simulink model "project_2023_12_11_P46"  (R2021b)
settings: Solver=ode5  StartTime=0.0  StopTime=500  FixedStep=0.01  RelTol=1e-3
values from neighbouring files (symbols this model uses):
  c1 = 1    [project_2023_12_11_P46_1.m]
  c2 = 1    [project_2023_12_11_P46_1.m]
  g = 9.8    [project_2023_12_11_P46_1.m]
  m = 70    [project_2023_12_11_P46_1.m]
undefined symbols (not defined in the file or in its folder): k
settings Model: Creator=Administrator  LastModifiedBy=yingguang wang
settings SolverCC: AlgebraicLoopSolver=TrustRegion
settings DataIOCC: SaveFormat=Array  ReturnWorkspaceOutputs=off  TimeSaveName=t  OutputSaveName=y
settings DebuggingCC: SFMachineParentedDataDiag=warning  ArithmeticOperatorsInVariantConditions=warning
settings SFSimCC: SimUseLocalCustomCode=off  CustomCodeUndefinedFunction=UseInterfaceOnly
settings RTWCC: RTWUseLocalCustomCode=off

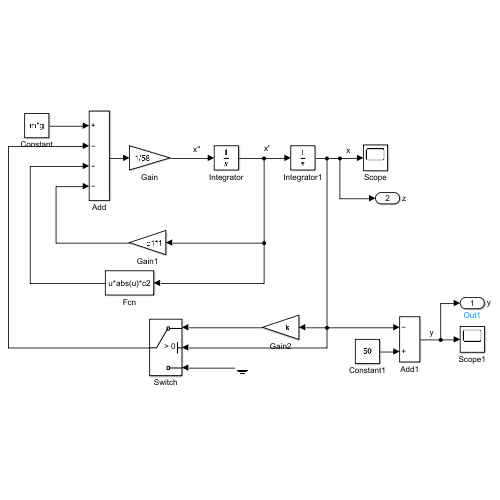
[thumbnail: Simulink's stored preview of the top-level diagram]
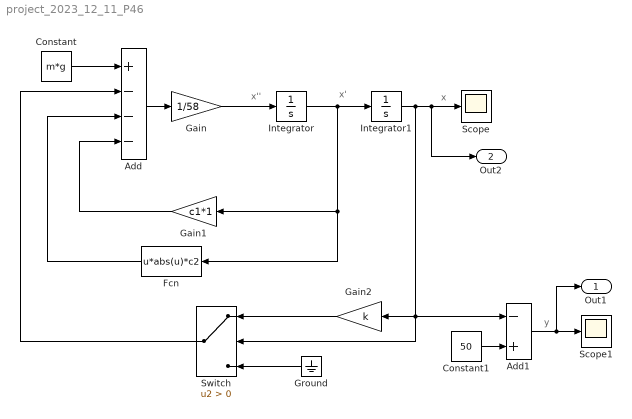
== system project_2023_12_11_P46 ==
  note: x'
  note: x''
  note: x
  note: y
  Add : Sum  Inputs=+---
  Add1 : Sum  Inputs=-+
  Constant : Constant  Value=m*g
  Constant1 : Constant  Value=50
  Fcn : Fcn  Expr=u*abs(u)*c2
  Gain : Gain  Gain=1/58
  Gain1 : Gain  Gain=c1*1
  Gain2 : Gain  Gain=k
  Ground : Ground
  Integrator : Integrator
  Integrator1 : Integrator  InitialCondition=-30
  Scope : Scope
  Scope1 : Scope
  Switch : Switch  Criteria=u2 > Threshold
  Out1 : Outport  SignalName=y  VectorParamsAs1DForOutWhenUnconnected=off
  Out2 : Outport  Port=2  SignalName=z  VectorParamsAs1DForOutWhenUnconnected=off
  wires:
  Constant/1 -> Add/1
  Add/1 -> Gain/1
  Gain/1 -> Integrator/1
  Integrator/1 -> Fcn/1, Gain1/1, Integrator1/1
  Fcn/1 -> Add/3
  Gain1/1 -> Add/4
  Switch/1 -> Add/2
  Gain2/1 -> Switch/1
  Ground/1 -> Switch/3
  Integrator1/1 -> Out2/1, Scope/1, Gain2/1, Add1/1, Switch/2
  Constant1/1 -> Add1/2
  Add1/1 -> Out1/1, Scope1/1
